simulink model "Rider_Controls_FullHarness"  (R2014b)
settings: Solver=FixedStepDiscrete  StartTime=0.0  StopTime=inf  RelTol=1e-3
PostLoadFcn:
  | load('Embedded_Config.mat')
model workspace: external: MAT-File Embedded_Config.mat (data not in the file)
undefined symbols (not defined in the file or in its folder): canChannel
libraries: canlib x3, canmsglib x2, realtime_pacer_lib x1
settings Model: Creator=The MathWorks Inc.  LastModifiedBy=Sean
settings DataIOCC: SignalLoggingSaveFormat=ModelDataLogs  SaveOutput=off  SaveTime=off
settings OptimizationCC: ExpressionDepthLimit=2147483647  InitFltsAndDblsToZero=on  OptimizeModelRefInitCode=on  LifeSpan=Inf  MaxStackSize=64
settings DebuggingCC: UnderspecifiedInitializationDetection=Classic  MergeDetectMultiDrivingBlocksExec=none  SignalResolutionControl=TryResolveAllWithWarning  SolverPrmCheckMsg=none  InheritedTsInSrcMsg=none  MultiTaskDSMMsg=warning  MultiTaskCondExecSysMsg=none  FcnCallInpInsideContextMsg=UseLocalSettings  StateNameClashWarn=warning
settings HardwareCC: ProdBitPerChar=16  ProdBitPerInt=16  ProdBitPerPointer=16  ProdLargestAtomicInteger=Integer  ProdIntDivRoundTo=Zero  ProdEndianess=LittleEndian  ProdWordSize=16  ProdHWDeviceType=Texas Instruments->C2000  TargetBitPerChar=16  TargetBitPerInt=16  TargetBitPerPointer=16  TargetLargestAtomicInteger=Integer  TargetIntDivRoundTo=Zero  TargetEndianess=LittleEndian  TargetWordSize=16  TargetHWDeviceType=Texas Instruments->C2000
settings RTWCC: SystemTargetFile=ert.tlc  TemplateMakefile=ert_default_tmf  PostCodeGenCommand=; ;codertarget.postCodeGenHookCommand(h)  Description=Embedded Coder  GenerateReport=on  ProcessScript=ert_make_rtw_hook  Toolchain=Texas Instruments Code Composer Studio v5 (C2000)  BuildConfiguration=Faster Runs  IncludeHyperlinkInReport=on  PortableWordSizes=on  CodeExecutionProfiling=on  CodeProfilingInstrumentation=on
settings CodeAppCC: IgnoreCustomStorageClasses=off  CustomSymbolStrType=$N$R$M  InternalIdentifier=Classic

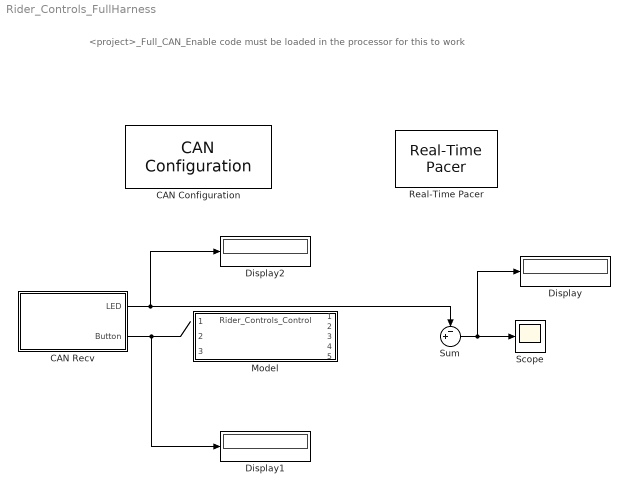
== system Rider_Controls_FullHarness ==
  note: <project>_Full_CAN_Enable code must be loaded
      | in the processor for this to work
  CAN Configuration : canlib/CAN Configuration  BlockHandle=2330.0011  DeviceMenu=Kvaser Virtual 1 (Channel 1)  Device=Kvaser Eagle 1 (Channel 1)  ObjConstructor=canChannel('Kvaser', 'Eagle 1', 1)  BusSpeed=500000  EnableBitParameters=off  SJW=1  TSEG1=4  TSEG2=3  NSamples=1  AckMode=Normal
  CAN Recv : Subsystem
  Display : Display
  Display1 : Display
  Display2 : Display
  Model : ModelReference  ModelNameDialog=Rider_Controls_Control.slx  SimulationMode=Normal  ModelReferenceVersion=1.108  CopyOfModelName=Rider_Controls_Control.slx  DefaultDataLogging=on
  Real-Time Pacer : realtime_pacer_lib/Real-Time Pacer  simTimePerRealTime=1
  Scope : Scope
  Sum : Sum  Inputs=-+|
  wires:
  CAN Recv/2(Button) -> Display1/1
  ? -> Sum/2
  CAN Recv/1(LED) -> Display2/1, Sum/1
  Sum/1 -> Display/1, Scope/1

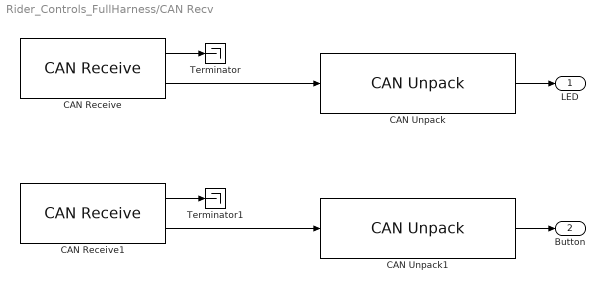
== system Rider_Controls_FullHarness/CAN Recv ==
  CAN Receive : canlib/CAN Receive  BlockHandle=3183.0038  DeviceMenu=Kvaser Eagle 1 (Channel 1)  Device=Kvaser Eagle 1 (Channel 1)  ObjConstructor=canChannel('Kvaser', 'Eagle 1', 1)  EnableStandardIDsFilter=off  StandardIDs=1  EnableExtendedIDsFilter=off  ExtendedIDs=0  SampleTime=.01  MsgsPerTimestep=all  StdIDsCombo=Allow only  ExtIDsCombo=Block all  InternalFilterUpdateStatus=on
  CAN Receive1 : canlib/CAN Receive  BlockHandle=3239.0011  DeviceMenu=Kvaser Eagle 1 (Channel 1)  Device=Kvaser Eagle 1 (Channel 1)  ObjConstructor=canChannel('Kvaser', 'Eagle 1', 1)  EnableStandardIDsFilter=off  StandardIDs=2  EnableExtendedIDsFilter=off  ExtendedIDs=0  SampleTime=.01  MsgsPerTimestep=all  StdIDsCombo=Allow only  ExtIDsCombo=Block all  InternalFilterUpdateStatus=on
  CAN Unpack : canmsglib/CAN Unpack  MsgList=(none)  MsgName=LED_Status  MsgIDType=Standard (11-bit identifier)  MsgIdentifier=1  MsgLength=2  SignalInfo=LED$0$16$1$1$1$0$1$0$-Inf$Inf$#  NSignals=1  IDPort=off  TimestampPort=off  ErrorPort=off  RemotePort=off  LengthPort=off  StatusPort=off  StartBits=str2num('[int32(0)]')  SignalSizes=str2num('[int32(16)]')  ByteOrders=str2num('[int32(1)]')  DataTypes=str2num('[int32(1)]')  MultiplexTypes=str2num('[int32(1)]')  MultiplexValues=str2num('[double(0)]')  Factors=str2num('[double(1)]')  Offsets=str2num('[double(0)]')  Minimums=str2num('[double(-Inf)]')  Maximums=str2num('[double(Inf)]')
  CAN Unpack1 : canmsglib/CAN Unpack  MsgList=(none)  MsgName=LED_Status  MsgIDType=Standard (11-bit identifier)  MsgIdentifier=2  MsgLength=2  SignalInfo=Button$0$16$1$1$1$0$1$0$-Inf$Inf$#  NSignals=1  IDPort=off  TimestampPort=off  ErrorPort=off  RemotePort=off  LengthPort=off  StatusPort=off  StartBits=str2num('[int32(0)]')  SignalSizes=str2num('[int32(16)]')  ByteOrders=str2num('[int32(1)]')  DataTypes=str2num('[int32(1)]')  MultiplexTypes=str2num('[int32(1)]')  MultiplexValues=str2num('[double(0)]')  Factors=str2num('[double(1)]')  Offsets=str2num('[double(0)]')  Minimums=str2num('[double(-Inf)]')  Maximums=str2num('[double(Inf)]')
  Terminator : Terminator
  Terminator1 : Terminator
  LED : Outport
  Button : Outport  Port=2
  wires:
  CAN Receive/1 -> Terminator/1
  CAN Receive/2 -> CAN Unpack/1
  CAN Unpack/1 -> LED/1
  CAN Receive1/1 -> Terminator1/1
  CAN Receive1/2 -> CAN Unpack1/1
  CAN Unpack1/1 -> Button/1
